simulink model "belt_traverse_control"  (R2022a)
settings: Solver=FixedStepAuto  StartTime=0.0  StopTime=inf  FixedStep=0.001  RelTol=1e-3
undefined symbols (not defined in the file): National_Instruments, PCIe
libraries: sldrtlib x10
settings Model: SimulationMode=external  Creator=xhe61  LastModifiedBy=ehandyca
settings HardwareCC: ProdBitPerLong=64  ProdHWDeviceType=Intel->x86-64 (Linux 64)
settings RTWCC: Description=Simulink Desktop Real-Time  SystemTargetFile=sldrt.tlc  TemplateMakefile=sldrt.tmf  RTWCompilerOptimization=on
settings CodeAppCC: MaxIdLength=95
settings SimulinkDesktopRealTimeCC: TargetLibSuffix=_sldrt.a  TargetPreCompLibLocation=C:\Program Files\MATLAB\R2022a\toolbox\sldrt\lib\win64

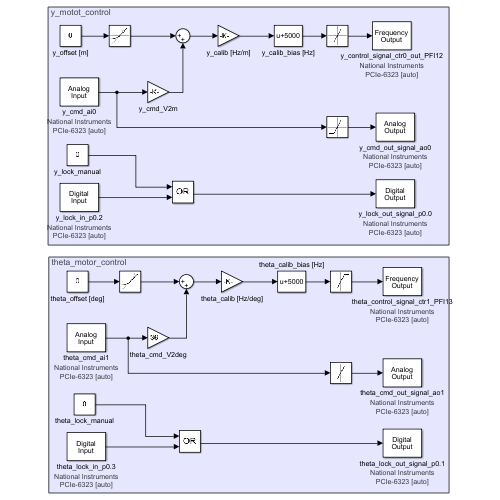
[thumbnail: Simulink's stored preview of the top-level diagram]
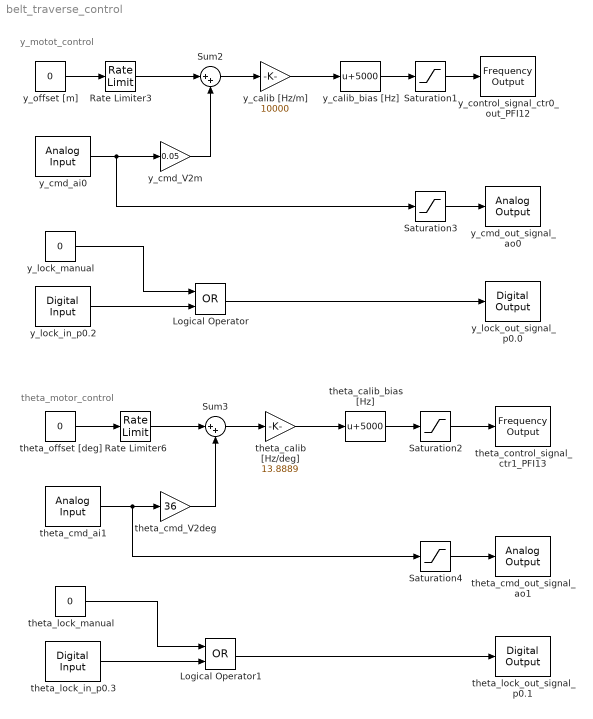
== system belt_traverse_control ==
  note: theta_motor_control
  note: y_motot_control
  Logical Operator : Logic  Operator=OR  AllPortsSameDT=off  OutDataTypeStr=boolean
  Logical Operator1 : Logic  Operator=OR  AllPortsSameDT=off  OutDataTypeStr=boolean
  Rate Limiter3 : RateLimiter  RisingSlewLimit=0.08  FallingSlewLimit=-0.08  SampleTimeMode=inherited
  Rate Limiter6 : RateLimiter  RisingSlewLimit=30  FallingSlewLimit=-30  SampleTimeMode=inherited
  Saturation1 : Saturate  UpperLimit=10000  LowerLimit=5000
  Saturation2 : Saturate  UpperLimit=10000  LowerLimit=5000
  Saturation3 : Saturate  UpperLimit=10  LowerLimit=-10
  Saturation4 : Saturate  UpperLimit=10  LowerLimit=-10
  Sum2 : Sum  Inputs=|++
  Sum3 : Sum  Inputs=|++
  theta_calib [Hz/deg] : Gain  Gain=13.8889
  theta_calib_bias [Hz] : Bias  Bias=5000  SaturateOnIntegerOverflow=off
  theta_cmd_V2deg : Gain  Gain=36
  theta_cmd_ai1 : sldrtlib/Analog Input  SampleTime=0.001  MaxMissedTicks=10  ShowMissedTicks=off  YieldWhenWaiting=off  DrvName=National_Instruments/PCIe-6323  DrvAddress=4294967295  DrvOptions=[0 3 61440 3 3 3 3]  Channels=2  RangeMode=1  VoltRange=1  DataType=1
      settings: AttributesFormatString=National Instruments\nPCIe-6323 [auto]
  theta_cmd_out_signal_ao1 : sldrtlib/Analog Output  SampleTime=0.001  MaxMissedTicks=10  ShowMissedTicks=off  YieldWhenWaiting=off  DrvName=National_Instruments/PCIe-6323  DrvAddress=4294967295  DrvOptions=[0 3 61440 3 3 3 3]  Channels=2  RangeMode=1  VoltRange=1  InitialValue=[]  FinalValue=[]
      settings: AttributesFormatString=National Instruments\nPCIe-6323 [auto]
  theta_control_signal_ctr1_PFI13 : sldrtlib/Frequency Output  SampleTime=0.001  MaxMissedTicks=10  ShowMissedTicks=off  YieldWhenWaiting=off  DrvName=National_Instruments/PCIe-6323  DrvAddress=4294967295  DrvOptions=[0 3 61440 3 3 3 3]  Channels=2  FrequencySource=2  Frequency=[]  FrequencyFinalValue=[]  DutySource=1  Duty=0.5  DutyFinalValue=[]
      settings: AttributesFormatString=National Instruments\nPCIe-6323 [auto]  SourceProductBaseCode=WT
  theta_lock_in_p0.3 : sldrtlib/Digital Input  SampleTime=0.001  MaxMissedTicks=10  ShowMissedTicks=off  YieldWhenWaiting=on  DrvName=National_Instruments/PCIe-6323  DrvAddress=4294967295  DrvOptions=[0 3 61440 3 3 3 3]  Channels=4  BitMode=1  DataType=9
      settings: AttributesFormatString=National Instruments\nPCIe-6323 [auto]  SourceProductBaseCode=WT
  theta_lock_manual : Constant  Value=0  OutDataTypeStr=boolean
  theta_lock_out_signal_p0.1 : sldrtlib/Digital Output  SampleTime=0.001  MaxMissedTicks=10  ShowMissedTicks=off  YieldWhenWaiting=off  DrvName=National_Instruments/PCIe-6323  DrvAddress=4294967295  DrvOptions=[0 3 61440 3 3 3 3]  Channels=1  BitMode=1  InitialValue=[]  FinalValue=[]
      settings: AttributesFormatString=National Instruments\nPCIe-6323 [auto]  SourceProductBaseCode=WT
  theta_offset [deg] : Constant  Value=0
  y_calib [Hz/m] : Gain  Gain=10000
  y_calib_bias [Hz] : Bias  Bias=5000  SaturateOnIntegerOverflow=off
  y_cmd_V2m : Gain  Gain=0.05
  y_cmd_ai0 : sldrtlib/Analog Input  SampleTime=0.001  MaxMissedTicks=10  ShowMissedTicks=off  YieldWhenWaiting=off  DrvName=National_Instruments/PCIe-6323  DrvAddress=4294967295  DrvOptions=[0 3 61440 3 3 3 3]  Channels=1  RangeMode=1  VoltRange=1  DataType=1
      settings: AttributesFormatString=National Instruments\nPCIe-6323 [auto]
  y_cmd_out_signal_ao0 : sldrtlib/Analog Output  SampleTime=0.001  MaxMissedTicks=10  ShowMissedTicks=off  YieldWhenWaiting=off  DrvName=National_Instruments/PCIe-6323  DrvAddress=4294967295  DrvOptions=[0 3 61440 3 3 3 3]  Channels=1  RangeMode=1  VoltRange=1  InitialValue=[]  FinalValue=[]
      settings: AttributesFormatString=National Instruments\nPCIe-6323 [auto]
  y_control_signal_ctr0_out_PFI12 : sldrtlib/Frequency Output  SampleTime=0.001  MaxMissedTicks=10  ShowMissedTicks=off  YieldWhenWaiting=off  DrvName=National_Instruments/PCIe-6323  DrvAddress=4294967295  DrvOptions=[0 3 61440 3 3 3 3]  Channels=1  FrequencySource=2  Frequency=[]  FrequencyFinalValue=[]  DutySource=1  Duty=0.5  DutyFinalValue=[]
      settings: AttributesFormatString=National Instruments\nPCIe-6323 [auto]  SourceProductBaseCode=WT
  y_lock_in_p0.2 : sldrtlib/Digital Input  SampleTime=0.001  MaxMissedTicks=10  ShowMissedTicks=off  YieldWhenWaiting=on  DrvName=National_Instruments/PCIe-6323  DrvAddress=4294967295  DrvOptions=[0 3 61440 3 3 3 3]  Channels=3  BitMode=1  DataType=9
      settings: AttributesFormatString=National Instruments\nPCIe-6323 [auto]  SourceProductBaseCode=WT
  y_lock_manual : Constant  Value=0  OutDataTypeStr=boolean
  y_lock_out_signal_p0.0 : sldrtlib/Digital Output  SampleTime=0.001  MaxMissedTicks=10  ShowMissedTicks=off  YieldWhenWaiting=off  DrvName=National_Instruments/PCIe-6323  DrvAddress=4294967295  DrvOptions=[0 3 61440 3 3 3 3]  Channels=1  BitMode=1  InitialValue=[]  FinalValue=[]
      settings: AttributesFormatString=National Instruments\nPCIe-6323 [auto]  SourceProductBaseCode=WT
  y_offset [m] : Constant  Value=0
  wires:
  y_offset [m]/1 -> Rate Limiter3/1
  y_calib [Hz/m]/1 -> y_calib_bias [Hz]/1
  y_calib_bias [Hz]/1 -> Saturation1/1
  Rate Limiter3/1 -> Sum2/1
  Saturation1/1 -> y_control_signal_ctr0_out_PFI12/1
  Sum2/1 -> y_calib [Hz/m]/1
  Sum3/1 -> theta_calib [Hz/deg]/1
  Rate Limiter6/1 -> Sum3/1
  theta_calib_bias [Hz]/1 -> Saturation2/1
  theta_offset [deg]/1 -> Rate Limiter6/1
  Saturation2/1 -> theta_control_signal_ctr1_PFI13/1
  theta_calib [Hz/deg]/1 -> theta_calib_bias [Hz]/1
  y_cmd_V2m/1 -> Sum2/2
  Saturation3/1 -> y_cmd_out_signal_ao0/1
  Saturation4/1 -> theta_cmd_out_signal_ao1/1
  theta_cmd_ai1/1 -> theta_cmd_V2deg/1, Saturation4/1
  theta_cmd_V2deg/1 -> Sum3/2
  y_cmd_ai0/1 -> Saturation3/1, y_cmd_V2m/1
  y_lock_manual/1 -> Logical Operator/1
  y_lock_in_p0.2/1 -> Logical Operator/2
  Logical Operator/1 -> y_lock_out_signal_p0.0/1
  theta_lock_manual/1 -> Logical Operator1/1
  theta_lock_in_p0.3/1 -> Logical Operator1/2
  Logical Operator1/1 -> theta_lock_out_signal_p0.1/1
